simulink model "TBS_SIM"  (R2021a)
settings: Solver=ode5  StartTime=15  StopTime=100  FixedStep=0.002  RelTol=1e-3
PreLoadFcn:
  | TBS_Cai_simu_init_20170316
StopFcn:
  | TBS_SIMULATION_LOG
undefined symbols (not defined in the file): air_density, g, L1X, L2X, L2Y, L3X, L3Y, MAC1, MAC2, MAC3, magnitude, mass, motor_m0, motor_t0, ORIGIN_CD, ORIGIN_CL, ORIGIN_CM, S_seg1, S_seg2, S_seg3
libraries: aerolibconvert2 x20, pid_lib x10, sharedtransform x4, aerolibwind2 x3, simulink x2, shared6dof x1, aerolibasang x1
(part 2 of 3)

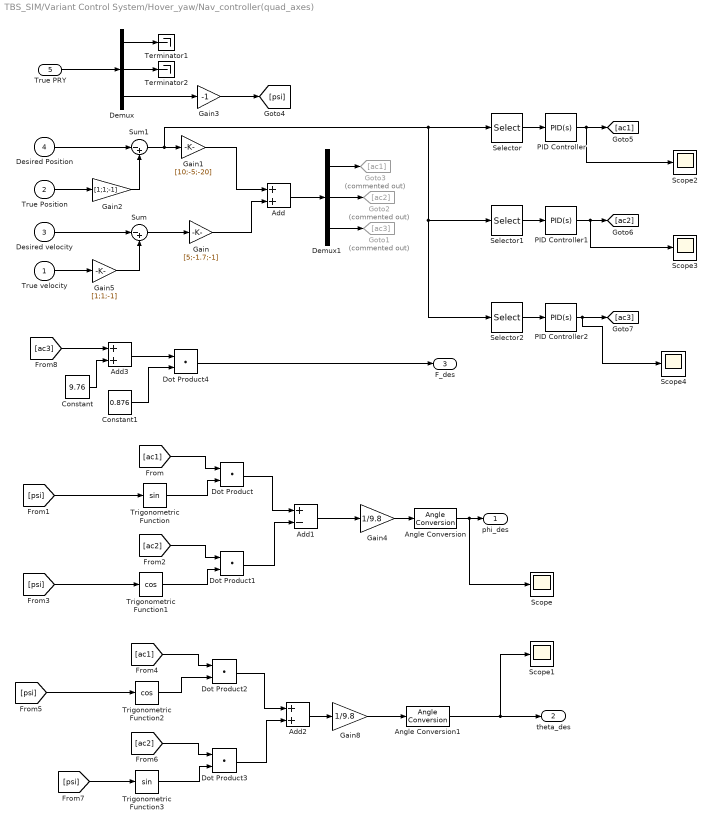
== system TBS_SIM/Variant Control System/Hover_yaw/Nav_controller(quad_axes) ==
  True velocity : Inport
  True Position : Inport  Port=2
  Desired velocity : Inport  Port=3
  Desired Position : Inport  Port=4
  True PRY : Inport  Port=5
  Add : Sum
  Add1 : Sum  Inputs=+-
  Add2 : Sum
  Add3 : Sum
  Angle Conversion : aerolibconvert2/Angle Conversion  IU=rad  OU=deg
  Angle Conversion1 : aerolibconvert2/Angle Conversion  IU=rad  OU=deg
  Constant : Constant  Value=9.76
  Constant1 : Constant  Value=0.876
  Demux : Demux  Outputs=3
  Demux1 : Demux  Outputs=3
  Dot Product{,1..4} (5 alike) : DotProduct  InputSameDT=on  OutDataTypeStr=Inherit: Inherit via internal rule
  Gain : Gain  Gain=[5;-1.7;-1]
  Gain1 : Gain  Gain=[10;-5;-20]
  Gain2 : Gain  Gain=[1;1;-1]
  Gain3 : Gain  Gain=-1
  Gain4 : Gain  Gain=1/9.8
  Gain5 : Gain  Gain=[1;1;-1]
  Gain8 : Gain  Gain=1/9.8
  Goto1 : Goto  Commented=on  GotoTag=ac3
  Goto2 : Goto  Commented=on  GotoTag=ac2
  Goto3 : Goto  Commented=on  GotoTag=ac1
  PID Controller : pid_lib/PID Controller  Controller=PID  Form=Parallel  TimeDomain=Continuous-time  UseExternalTs=off  SampleTime=-1  IntegratorMethod=Forward Euler  FilterMethod=Forward Euler  ControllerParametersSource=internal  P=4  I=3  D=3  UseFilter=on  N=100  TunerSelectOption=Transfer Function Based (PID Tuner App)  InitialConditionSource=internal  InitialConditionForIntegrator=0  InitialConditionForFilter=0  DifferentiatorICPrevScaledInput=0  ExternalReset=none  TrackingMode=off  Kt=1  LimitOutput=off  SatLimitsSource=internal  UpperSaturationLimit=inf  LowerSaturationLimit=-inf  LinearizeAsGain=on  AntiWindupMode=none  Kb=1  POutMin=[]  POutMax=[]  IOutMin=[]  IOutMax=[]  DOutMin=[]  DOutMax=[]  NOutMin=[]  NOutMax=[]  SumOutMin=[]  SumOutMax=[]  SaturationOutMin=[]  SaturationOutMax=[]  PParamMin=[]  PParamMax=[]  IParamMin=[]  IParamMax=[]  DParamMin=[]  DParamMax=[]  NParamMin=[]  NParamMax=[]  KbParamMin=[]  KbParamMax=[]  KtParamMin=[]  KtParamMax=[]  KbOutMin=[]  KbOutMax=[]  KtOutMin=[]  KtOutMax=[]  IntegratorOutMin=[]  IntegratorOutMax=[]  FilterOutMin=[]  FilterOutMax=[]  SumI1OutMin=[]  SumI1OutMax=[]  SumI2OutMin=[]  SumI2OutMax=[]  SumI3OutMin=[]  SumI3OutMax=[]  SumI4OutMin=[]  SumI4OutMax=[]  SumDOutMin=[]  SumDOutMax=[]  DifferentiatorOutMin=[]  DifferentiatorOutMax=[]  FilterDiffOutCoefMin=[]  FilterDiffOutCoefMax=[]  ReciprocalOutMin=[]  ReciprocalOutMax=[]  SumDenOutMin=[]  SumDenOutMax=[]  SumNumOutMin=[]  SumNumOutMax=[]  DivideOutMin=[]  DivideOutMax=[]  UdiffTsProdOutMin=[]  UdiffTsProdOutMax=[]  NTsProdOutMin=[]  NTsProdOutMax=[]  UintegralTsProdOutMin=[]  UintegralTsProdOutMax=[]  UngainTsProdOutMin=[]  UngainTsProdOutMax=[]  IntegratorContinuousStateAttributes=''  IntegratorStateMustResolveToSignalObject=off  IntegratorRTWStateStorageClass=Auto  FilterContinuousStateAttributes=''  FilterStateMustResolveToSignalObject=off  FilterRTWStateStorageClass=Auto  ParallelPVariant=InternalParameters  IdealPVariant=Disabled  IVariant=InternalParameters  DVariant=InternalParameters  IntegratorVariant=Continuous  SatVariant=Disabled  AWVariant=Passthrough  PCopyVariant=Disabled  TRVariant=Disabled  FdbkBlocksVariant=Forward  IdealPFdbkVariant=Disabled  SatFdbkVariant=Disabled  DerivativeFilterVariant=ContFilter  NVariant=InternalParameters  NCopyVariant=Disabled  FilterICVariant=InternalICsFilter  IntegratorICVariant=InternalICs  ExternalResetVariant=Disabled  TRSumVariant=Passthrough  SumFdbkVariant=Disabled  SumVariant=Sum_PID  TsampFilterVariant=InternalTs  TsampNgainVariant=Passthrough  TsampIntegralVariant=Passthrough  ExternalSaturationOutDataTypeStr=Inherit: Same as second input
  PID Controller1 : pid_lib/PID Controller  Controller=PID  Form=Parallel  TimeDomain=Continuous-time  UseExternalTs=off  SampleTime=-1  IntegratorMethod=Forward Euler  FilterMethod=Forward Euler  ControllerParametersSource=internal  P=-8  I=-4  D=-2  UseFilter=on  N=100  TunerSelectOption=Transfer Function Based (PID Tuner App)  InitialConditionSource=internal  InitialConditionForIntegrator=0  InitialConditionForFilter=0  DifferentiatorICPrevScaledInput=0  ExternalReset=none  TrackingMode=off  Kt=1  LimitOutput=off  SatLimitsSource=internal  UpperSaturationLimit=inf  LowerSaturationLimit=-inf  LinearizeAsGain=on  AntiWindupMode=none  Kb=1  POutMin=[]  POutMax=[]  IOutMin=[]  IOutMax=[]  DOutMin=[]  DOutMax=[]  NOutMin=[]  NOutMax=[]  SumOutMin=[]  SumOutMax=[]  SaturationOutMin=[]  SaturationOutMax=[]  PParamMin=[]  PParamMax=[]  IParamMin=[]  IParamMax=[]  DParamMin=[]  DParamMax=[]  NParamMin=[]  NParamMax=[]  KbParamMin=[]  KbParamMax=[]  KtParamMin=[]  KtParamMax=[]  KbOutMin=[]  KbOutMax=[]  KtOutMin=[]  KtOutMax=[]  IntegratorOutMin=[]  IntegratorOutMax=[]  FilterOutMin=[]  FilterOutMax=[]  SumI1OutMin=[]  SumI1OutMax=[]  SumI2OutMin=[]  SumI2OutMax=[]  SumI3OutMin=[]  SumI3OutMax=[]  SumI4OutMin=[]  SumI4OutMax=[]  SumDOutMin=[]  SumDOutMax=[]  DifferentiatorOutMin=[]  DifferentiatorOutMax=[]  FilterDiffOutCoefMin=[]  FilterDiffOutCoefMax=[]  ReciprocalOutMin=[]  ReciprocalOutMax=[]  SumDenOutMin=[]  SumDenOutMax=[]  SumNumOutMin=[]  SumNumOutMax=[]  DivideOutMin=[]  DivideOutMax=[]  UdiffTsProdOutMin=[]  UdiffTsProdOutMax=[]  NTsProdOutMin=[]  NTsProdOutMax=[]  UintegralTsProdOutMin=[]  UintegralTsProdOutMax=[]  UngainTsProdOutMin=[]  UngainTsProdOutMax=[]  IntegratorContinuousStateAttributes=''  IntegratorStateMustResolveToSignalObject=off  IntegratorRTWStateStorageClass=Auto  FilterContinuousStateAttributes=''  FilterStateMustResolveToSignalObject=off  FilterRTWStateStorageClass=Auto  ParallelPVariant=InternalParameters  IdealPVariant=Disabled  IVariant=InternalParameters  DVariant=InternalParameters  IntegratorVariant=Continuous  SatVariant=Disabled  AWVariant=Passthrough  PCopyVariant=Disabled  TRVariant=Disabled  FdbkBlocksVariant=Forward  IdealPFdbkVariant=Disabled  SatFdbkVariant=Disabled  DerivativeFilterVariant=ContFilter  NVariant=InternalParameters  NCopyVariant=Disabled  FilterICVariant=InternalICsFilter  IntegratorICVariant=InternalICs  ExternalResetVariant=Disabled  TRSumVariant=Passthrough  SumFdbkVariant=Disabled  SumVariant=Sum_PID  TsampFilterVariant=InternalTs  TsampNgainVariant=Passthrough  TsampIntegralVariant=Passthrough  ExternalSaturationOutDataTypeStr=Inherit: Same as second input
  PID Controller2 : pid_lib/PID Controller  Controller=PID  Form=Parallel  TimeDomain=Continuous-time  UseExternalTs=off  SampleTime=-1  IntegratorMethod=Forward Euler  FilterMethod=Forward Euler  ControllerParametersSource=internal  P=-9  I=-5  D=-2  UseFilter=on  N=100  TunerSelectOption=Transfer Function Based (PID Tuner App)  InitialConditionSource=internal  InitialConditionForIntegrator=0  InitialConditionForFilter=0  DifferentiatorICPrevScaledInput=0  ExternalReset=none  TrackingMode=off  Kt=1  LimitOutput=off  SatLimitsSource=internal  UpperSaturationLimit=inf  LowerSaturationLimit=-inf  LinearizeAsGain=on  AntiWindupMode=none  Kb=1  POutMin=[]  POutMax=[]  IOutMin=[]  IOutMax=[]  DOutMin=[]  DOutMax=[]  NOutMin=[]  NOutMax=[]  SumOutMin=[]  SumOutMax=[]  SaturationOutMin=[]  SaturationOutMax=[]  PParamMin=[]  PParamMax=[]  IParamMin=[]  IParamMax=[]  DParamMin=[]  DParamMax=[]  NParamMin=[]  NParamMax=[]  KbParamMin=[]  KbParamMax=[]  KtParamMin=[]  KtParamMax=[]  KbOutMin=[]  KbOutMax=[]  KtOutMin=[]  KtOutMax=[]  IntegratorOutMin=[]  IntegratorOutMax=[]  FilterOutMin=[]  FilterOutMax=[]  SumI1OutMin=[]  SumI1OutMax=[]  SumI2OutMin=[]  SumI2OutMax=[]  SumI3OutMin=[]  SumI3OutMax=[]  SumI4OutMin=[]  SumI4OutMax=[]  SumDOutMin=[]  SumDOutMax=[]  DifferentiatorOutMin=[]  DifferentiatorOutMax=[]  FilterDiffOutCoefMin=[]  FilterDiffOutCoefMax=[]  ReciprocalOutMin=[]  ReciprocalOutMax=[]  SumDenOutMin=[]  SumDenOutMax=[]  SumNumOutMin=[]  SumNumOutMax=[]  DivideOutMin=[]  DivideOutMax=[]  UdiffTsProdOutMin=[]  UdiffTsProdOutMax=[]  NTsProdOutMin=[]  NTsProdOutMax=[]  UintegralTsProdOutMin=[]  UintegralTsProdOutMax=[]  UngainTsProdOutMin=[]  UngainTsProdOutMax=[]  IntegratorContinuousStateAttributes=''  IntegratorStateMustResolveToSignalObject=off  IntegratorRTWStateStorageClass=Auto  FilterContinuousStateAttributes=''  FilterStateMustResolveToSignalObject=off  FilterRTWStateStorageClass=Auto  ParallelPVariant=InternalParameters  IdealPVariant=Disabled  IVariant=InternalParameters  DVariant=InternalParameters  IntegratorVariant=Continuous  SatVariant=Disabled  AWVariant=Passthrough  PCopyVariant=Disabled  TRVariant=Disabled  FdbkBlocksVariant=Forward  IdealPFdbkVariant=Disabled  SatFdbkVariant=Disabled  DerivativeFilterVariant=ContFilter  NVariant=InternalParameters  NCopyVariant=Disabled  FilterICVariant=InternalICsFilter  IntegratorICVariant=InternalICs  ExternalResetVariant=Disabled  TRSumVariant=Passthrough  SumFdbkVariant=Disabled  SumVariant=Sum_PID  TsampFilterVariant=InternalTs  TsampNgainVariant=Passthrough  TsampIntegralVariant=Passthrough  ExternalSaturationOutDataTypeStr=Inherit: Same as second input
  Scope{,1..4} (5 alike) : Scope
  Selector : Selector  InputPortWidth=3  IndexOptions=Index vector (dialog)  Indices=[1]  OutputSizes=1
  Selector1 : Selector  InputPortWidth=3  IndexOptions=Index vector (dialog)  Indices=[2]  OutputSizes=1
  Selector2 : Selector  InputPortWidth=3  IndexOptions=Index vector (dialog)  Indices=[3]  OutputSizes=1
  Sum : Sum  Inputs=|-+
  Sum1 : Sum  Inputs=|-+
  Terminator1 : Terminator
  Terminator2 : Terminator
  Trigonometric Function : Trigonometry
  Trigonometric Function1 : Trigonometry  Operator=cos
  Trigonometric Function2 : Trigonometry  Operator=cos
  Trigonometric Function3 : Trigonometry
  phi_des : Outport
  "theta_des " : Outport  Port=2
  F_des : Outport  Port=3
  wires:
  True velocity/1 -> Gain5/1
  Desired velocity/1 -> Sum/1
  Sum/1 -> Gain/1
  Gain1/1 -> Add/1
  Gain/1 -> Add/2
  True PRY/1 -> Demux/1
  Demux/1 -> Terminator1/1
  Demux/3 -> Gain3/1
  Demux/2 -> Terminator2/1
  Add/1 -> Demux1/1
  Demux1/2 -> Goto2/1
  [ac1] -> Dot Product/1
  Trigonometric Function/1 -> Dot Product/2
  [psi] -> Trigonometric Function/1
  [ac2] -> Dot Product1/1
  Trigonometric Function1/1 -> Dot Product1/2
  [psi] -> Trigonometric Function1/1
  Dot Product/1 -> Add1/1
  Dot Product1/1 -> Add1/2
  Add1/1 -> Gain4/1
  [ac1] -> Dot Product2/1
  Trigonometric Function2/1 -> Dot Product2/2
  [psi] -> Trigonometric Function2/1
  [ac2] -> Dot Product3/1
  Trigonometric Function3/1 -> Dot Product3/2
  [psi] -> Trigonometric Function3/1
  Dot Product2/1 -> Add2/1
  Dot Product3/1 -> Add2/2
  Add2/1 -> Gain8/1
  [ac3] -> Add3/1
  Constant/1 -> Add3/2
  Add3/1 -> Dot Product4/1
  Constant1/1 -> Dot Product4/2
  Dot Product4/1 -> F_des/1
  Demux1/1 -> Goto3/1
  Demux1/3 -> Goto1/1
  True Position/1 -> Gain2/1
  Gain2/1 -> Sum1/2
  Desired Position/1 -> Sum1/1
  Gain3/1 -> [psi]
  Gain4/1 -> Angle Conversion/1
  Angle Conversion/1 -> Scope/1, phi_des/1
  Gain8/1 -> Angle Conversion1/1
  Angle Conversion1/1 -> Scope1/1, "theta_des "/1
  Gain5/1 -> Sum/2
  Selector/1 -> PID Controller/1
  PID Controller/1 -> Scope2/1, [ac1]
  Selector1/1 -> PID Controller1/1
  PID Controller1/1 -> Scope3/1, [ac2]
  Sum1/1 -> Selector2/1, Selector1/1, Selector/1, Gain1/1
  Selector2/1 -> PID Controller2/1
  PID Controller2/1 -> Scope4/1, [ac3]

== system TBS_SIM/Variant Control System/Hover_yaw/map1 ==
  F_c : Inport
  M_c : Inport  Port=2
  Constant : Constant  Value=100
  Constant1 : Constant  Value=9.5
  Constant2 : Constant  Value=0.3
  Demux : Demux  Outputs=3
  Gain : Gain  Gain=1000
  Gain1 : Gain  Gain=1000
  Gain2 : Gain  Gain=50
  Gain3 : Gain  Gain=50
  Mux : Mux
  Sum : Sum  Inputs=-+|
  Sum1 : Sum  Inputs=|++
  Sum2 : Sum  Inputs=|+-
  Sum3 : Sum  Inputs=-+|
  Sum4 : Sum  Inputs=|++
  Sum5 : Sum  Inputs=|++
  Sum6 : Sum  Inputs=+-|
  Act : Outport
  wires:
  M_c/1 -> Demux/1
  F_c/1 -> Gain/1
  Demux/1 -> Gain1/1
  Gain1/1 -> Sum/2
  Constant/1 -> Sum/1
  Gain/1 -> Sum2/1, Sum1/1
  Sum/1 -> Sum1/2, Sum2/2
  Sum1/1 -> Mux/1
  Sum2/1 -> Mux/2
  Demux/2 -> Gain2/1
  Demux/3 -> Gain3/1
  Gain3/1 -> Sum4/1
  Constant1/1 -> Sum3/1
  Gain2/1 -> Sum3/2
  Constant2/1 -> Sum4/2
  Mux/1 -> Act/1
  Sum3/1 -> Sum5/1
  Sum4/1 -> Sum6/2, Sum5/2
  Sum5/1 -> Mux/4, Sum6/1
  Sum6/1 -> Mux/3

== system TBS_SIM/Variant Control System/PIDcruise/Subsystem ==
  Euler : Inport
  Constant : Constant  Value=0
  Constant1 : Constant  Value=8
  Constant2 : Constant  Value=0
  Demux : Demux  Outputs=3
  Mux : Mux  Inputs=3
  PID Controller : pid_lib/PID Controller  Controller=PID  Form=Parallel  TimeDomain=Continuous-time  UseExternalTs=off  SampleTime=-1  IntegratorMethod=Forward Euler  FilterMethod=Forward Euler  ControllerParametersSource=internal  P=0.5  I=0.1  D=0.01  UseFilter=on  N=100  TunerSelectOption=Transfer Function Based (PID Tuner App)  InitialConditionSource=internal  InitialConditionForIntegrator=0  InitialConditionForFilter=0  DifferentiatorICPrevScaledInput=0  ExternalReset=none  TrackingMode=off  Kt=1  LimitOutput=off  SatLimitsSource=internal  UpperSaturationLimit=inf  LowerSaturationLimit=-inf  LinearizeAsGain=on  AntiWindupMode=none  Kb=1  POutMin=[]  POutMax=[]  IOutMin=[]  IOutMax=[]  DOutMin=[]  DOutMax=[]  NOutMin=[]  NOutMax=[]  SumOutMin=[]  SumOutMax=[]  SaturationOutMin=[]  SaturationOutMax=[]  PParamMin=[]  PParamMax=[]  IParamMin=[]  IParamMax=[]  DParamMin=[]  DParamMax=[]  NParamMin=[]  NParamMax=[]  KbParamMin=[]  KbParamMax=[]  KtParamMin=[]  KtParamMax=[]  KbOutMin=[]  KbOutMax=[]  KtOutMin=[]  KtOutMax=[]  IntegratorOutMin=[]  IntegratorOutMax=[]  FilterOutMin=[]  FilterOutMax=[]  SumI1OutMin=[]  SumI1OutMax=[]  SumI2OutMin=[]  SumI2OutMax=[]  SumI3OutMin=[]  SumI3OutMax=[]  SumI4OutMin=[]  SumI4OutMax=[]  SumDOutMin=[]  SumDOutMax=[]  DifferentiatorOutMin=[]  DifferentiatorOutMax=[]  FilterDiffOutCoefMin=[]  FilterDiffOutCoefMax=[]  ReciprocalOutMin=[]  ReciprocalOutMax=[]  SumDenOutMin=[]  SumDenOutMax=[]  SumNumOutMin=[]  SumNumOutMax=[]  DivideOutMin=[]  DivideOutMax=[]  UdiffTsProdOutMin=[]  UdiffTsProdOutMax=[]  NTsProdOutMin=[]  NTsProdOutMax=[]  UintegralTsProdOutMin=[]  UintegralTsProdOutMax=[]  UngainTsProdOutMin=[]  UngainTsProdOutMax=[]  IntegratorContinuousStateAttributes=''  IntegratorStateMustResolveToSignalObject=off  IntegratorRTWStateStorageClass=Auto  FilterContinuousStateAttributes=''  FilterStateMustResolveToSignalObject=off  FilterRTWStateStorageClass=Auto  ParallelPVariant=InternalParameters  IdealPVariant=Disabled  IVariant=InternalParameters  DVariant=InternalParameters  IntegratorVariant=Continuous  SatVariant=Disabled  AWVariant=Passthrough  PCopyVariant=Disabled  TRVariant=Disabled  FdbkBlocksVariant=Forward  IdealPFdbkVariant=Disabled  SatFdbkVariant=Disabled  DerivativeFilterVariant=ContFilter  NVariant=InternalParameters  NCopyVariant=Disabled  FilterICVariant=InternalICsFilter  IntegratorICVariant=InternalICs  ExternalResetVariant=Disabled  TRSumVariant=Passthrough  SumFdbkVariant=Disabled  SumVariant=Sum_PID  TsampFilterVariant=InternalTs  TsampNgainVariant=Passthrough  TsampIntegralVariant=Passthrough  ExternalSaturationOutDataTypeStr=Inherit: Same as second input
  PID Controller1 : pid_lib/PID Controller  Controller=PID  Form=Parallel  TimeDomain=Continuous-time  UseExternalTs=off  SampleTime=-1  IntegratorMethod=Forward Euler  FilterMethod=Forward Euler  ControllerParametersSource=internal  P=0.8  I=0.5  D=0.005  UseFilter=on  N=100  TunerSelectOption=Transfer Function Based (PID Tuner App)  InitialConditionSource=internal  InitialConditionForIntegrator=0  InitialConditionForFilter=0  DifferentiatorICPrevScaledInput=0  ExternalReset=none  TrackingMode=off  Kt=1  LimitOutput=off  SatLimitsSource=internal  UpperSaturationLimit=inf  LowerSaturationLimit=-inf  LinearizeAsGain=on  AntiWindupMode=none  Kb=1  POutMin=[]  POutMax=[]  IOutMin=[]  IOutMax=[]  DOutMin=[]  DOutMax=[]  NOutMin=[]  NOutMax=[]  SumOutMin=[]  SumOutMax=[]  SaturationOutMin=[]  SaturationOutMax=[]  PParamMin=[]  PParamMax=[]  IParamMin=[]  IParamMax=[]  DParamMin=[]  DParamMax=[]  NParamMin=[]  NParamMax=[]  KbParamMin=[]  KbParamMax=[]  KtParamMin=[]  KtParamMax=[]  KbOutMin=[]  KbOutMax=[]  KtOutMin=[]  KtOutMax=[]  IntegratorOutMin=[]  IntegratorOutMax=[]  FilterOutMin=[]  FilterOutMax=[]  SumI1OutMin=[]  SumI1OutMax=[]  SumI2OutMin=[]  SumI2OutMax=[]  SumI3OutMin=[]  SumI3OutMax=[]  SumI4OutMin=[]  SumI4OutMax=[]  SumDOutMin=[]  SumDOutMax=[]  DifferentiatorOutMin=[]  DifferentiatorOutMax=[]  FilterDiffOutCoefMin=[]  FilterDiffOutCoefMax=[]  ReciprocalOutMin=[]  ReciprocalOutMax=[]  SumDenOutMin=[]  SumDenOutMax=[]  SumNumOutMin=[]  SumNumOutMax=[]  DivideOutMin=[]  DivideOutMax=[]  UdiffTsProdOutMin=[]  UdiffTsProdOutMax=[]  NTsProdOutMin=[]  NTsProdOutMax=[]  UintegralTsProdOutMin=[]  UintegralTsProdOutMax=[]  UngainTsProdOutMin=[]  UngainTsProdOutMax=[]  IntegratorContinuousStateAttributes=''  IntegratorStateMustResolveToSignalObject=off  IntegratorRTWStateStorageClass=Auto  FilterContinuousStateAttributes=''  FilterStateMustResolveToSignalObject=off  FilterRTWStateStorageClass=Auto  ParallelPVariant=InternalParameters  IdealPVariant=Disabled  IVariant=InternalParameters  DVariant=InternalParameters  IntegratorVariant=Continuous  SatVariant=Disabled  AWVariant=Passthrough  PCopyVariant=Disabled  TRVariant=Disabled  FdbkBlocksVariant=Forward  IdealPFdbkVariant=Disabled  SatFdbkVariant=Disabled  DerivativeFilterVariant=ContFilter  NVariant=InternalParameters  NCopyVariant=Disabled  FilterICVariant=InternalICsFilter  IntegratorICVariant=InternalICs  ExternalResetVariant=Disabled  TRSumVariant=Passthrough  SumFdbkVariant=Disabled  SumVariant=Sum_PID  TsampFilterVariant=InternalTs  TsampNgainVariant=Passthrough  TsampIntegralVariant=Passthrough  ExternalSaturationOutDataTypeStr=Inherit: Same as second input
  PID Controller2 : pid_lib/PID Controller  Controller=PID  Form=Parallel  TimeDomain=Continuous-time  UseExternalTs=off  SampleTime=-1  IntegratorMethod=Forward Euler  FilterMethod=Forward Euler  ControllerParametersSource=internal  P=3  I=1.5  D=0.5  UseFilter=on  N=100  TunerSelectOption=Transfer Function Based (PID Tuner App)  InitialConditionSource=internal  InitialConditionForIntegrator=0  InitialConditionForFilter=0  DifferentiatorICPrevScaledInput=0  ExternalReset=none  TrackingMode=off  Kt=1  LimitOutput=off  SatLimitsSource=internal  UpperSaturationLimit=inf  LowerSaturationLimit=-inf  LinearizeAsGain=on  AntiWindupMode=none  Kb=1  POutMin=[]  POutMax=[]  IOutMin=[]  IOutMax=[]  DOutMin=[]  DOutMax=[]  NOutMin=[]  NOutMax=[]  SumOutMin=[]  SumOutMax=[]  SaturationOutMin=[]  SaturationOutMax=[]  PParamMin=[]  PParamMax=[]  IParamMin=[]  IParamMax=[]  DParamMin=[]  DParamMax=[]  NParamMin=[]  NParamMax=[]  KbParamMin=[]  KbParamMax=[]  KtParamMin=[]  KtParamMax=[]  KbOutMin=[]  KbOutMax=[]  KtOutMin=[]  KtOutMax=[]  IntegratorOutMin=[]  IntegratorOutMax=[]  FilterOutMin=[]  FilterOutMax=[]  SumI1OutMin=[]  SumI1OutMax=[]  SumI2OutMin=[]  SumI2OutMax=[]  SumI3OutMin=[]  SumI3OutMax=[]  SumI4OutMin=[]  SumI4OutMax=[]  SumDOutMin=[]  SumDOutMax=[]  DifferentiatorOutMin=[]  DifferentiatorOutMax=[]  FilterDiffOutCoefMin=[]  FilterDiffOutCoefMax=[]  ReciprocalOutMin=[]  ReciprocalOutMax=[]  SumDenOutMin=[]  SumDenOutMax=[]  SumNumOutMin=[]  SumNumOutMax=[]  DivideOutMin=[]  DivideOutMax=[]  UdiffTsProdOutMin=[]  UdiffTsProdOutMax=[]  NTsProdOutMin=[]  NTsProdOutMax=[]  UintegralTsProdOutMin=[]  UintegralTsProdOutMax=[]  UngainTsProdOutMin=[]  UngainTsProdOutMax=[]  IntegratorContinuousStateAttributes=''  IntegratorStateMustResolveToSignalObject=off  IntegratorRTWStateStorageClass=Auto  FilterContinuousStateAttributes=''  FilterStateMustResolveToSignalObject=off  FilterRTWStateStorageClass=Auto  ParallelPVariant=InternalParameters  IdealPVariant=Disabled  IVariant=InternalParameters  DVariant=InternalParameters  IntegratorVariant=Continuous  SatVariant=Disabled  AWVariant=Passthrough  PCopyVariant=Disabled  TRVariant=Disabled  FdbkBlocksVariant=Forward  IdealPFdbkVariant=Disabled  SatFdbkVariant=Disabled  DerivativeFilterVariant=ContFilter  NVariant=InternalParameters  NCopyVariant=Disabled  FilterICVariant=InternalICsFilter  IntegratorICVariant=InternalICs  ExternalResetVariant=Disabled  TRSumVariant=Passthrough  SumFdbkVariant=Disabled  SumVariant=Sum_PID  TsampFilterVariant=InternalTs  TsampNgainVariant=Passthrough  TsampIntegralVariant=Passthrough  ExternalSaturationOutDataTypeStr=Inherit: Same as second input
  Sum : Sum  Inputs=+-|
  Sum1 : Sum  Inputs=+-|
  Sum2 : Sum  Inputs=+-|
  Out1 : Outport
  wires:
  Euler/1 -> Demux/1
  Sum/1 -> PID Controller/1
  Demux/1 -> Sum/2
  Constant/1 -> Sum/1
  Sum1/1 -> PID Controller1/1
  Demux/2 -> Sum1/2
  Constant1/1 -> Sum1/1
  Sum2/1 -> PID Controller2/1
  Demux/3 -> Sum2/2
  Constant2/1 -> Sum2/1
  PID Controller/1 -> Mux/1
  PID Controller1/1 -> Mux/2
  PID Controller2/1 -> Mux/3
  Mux/1 -> Out1/1

== system TBS_SIM/Variant Control System/PIDcruise/Subsystem1 ==
  Velocity : Inport
  Constant : Constant  Value=10
  PID Controller2 : pid_lib/PID Controller  Controller=PID  Form=Parallel  TimeDomain=Continuous-time  UseExternalTs=off  SampleTime=-1  IntegratorMethod=Forward Euler  FilterMethod=Forward Euler  ControllerParametersSource=internal  P=3  I=1  D=0.5  UseFilter=on  N=100  TunerSelectOption=Transfer Function Based (PID Tuner App)  InitialConditionSource=internal  InitialConditionForIntegrator=0  InitialConditionForFilter=0  DifferentiatorICPrevScaledInput=0  ExternalReset=none  TrackingMode=off  Kt=1  LimitOutput=off  SatLimitsSource=internal  UpperSaturationLimit=inf  LowerSaturationLimit=-inf  LinearizeAsGain=on  AntiWindupMode=none  Kb=1  POutMin=[]  POutMax=[]  IOutMin=[]  IOutMax=[]  DOutMin=[]  DOutMax=[]  NOutMin=[]  NOutMax=[]  SumOutMin=[]  SumOutMax=[]  SaturationOutMin=[]  SaturationOutMax=[]  PParamMin=[]  PParamMax=[]  IParamMin=[]  IParamMax=[]  DParamMin=[]  DParamMax=[]  NParamMin=[]  NParamMax=[]  KbParamMin=[]  KbParamMax=[]  KtParamMin=[]  KtParamMax=[]  KbOutMin=[]  KbOutMax=[]  KtOutMin=[]  KtOutMax=[]  IntegratorOutMin=[]  IntegratorOutMax=[]  FilterOutMin=[]  FilterOutMax=[]  SumI1OutMin=[]  SumI1OutMax=[]  SumI2OutMin=[]  SumI2OutMax=[]  SumI3OutMin=[]  SumI3OutMax=[]  SumI4OutMin=[]  SumI4OutMax=[]  SumDOutMin=[]  SumDOutMax=[]  DifferentiatorOutMin=[]  DifferentiatorOutMax=[]  FilterDiffOutCoefMin=[]  FilterDiffOutCoefMax=[]  ReciprocalOutMin=[]  ReciprocalOutMax=[]  SumDenOutMin=[]  SumDenOutMax=[]  SumNumOutMin=[]  SumNumOutMax=[]  DivideOutMin=[]  DivideOutMax=[]  UdiffTsProdOutMin=[]  UdiffTsProdOutMax=[]  NTsProdOutMin=[]  NTsProdOutMax=[]  UintegralTsProdOutMin=[]  UintegralTsProdOutMax=[]  UngainTsProdOutMin=[]  UngainTsProdOutMax=[]  IntegratorContinuousStateAttributes=''  IntegratorStateMustResolveToSignalObject=off  IntegratorRTWStateStorageClass=Auto  FilterContinuousStateAttributes=''  FilterStateMustResolveToSignalObject=off  FilterRTWStateStorageClass=Auto  ParallelPVariant=InternalParameters  IdealPVariant=Disabled  IVariant=InternalParameters  DVariant=InternalParameters  IntegratorVariant=Continuous  SatVariant=Disabled  AWVariant=Passthrough  PCopyVariant=Disabled  TRVariant=Disabled  FdbkBlocksVariant=Forward  IdealPFdbkVariant=Disabled  SatFdbkVariant=Disabled  DerivativeFilterVariant=ContFilter  NVariant=InternalParameters  NCopyVariant=Disabled  FilterICVariant=InternalICsFilter  IntegratorICVariant=InternalICs  ExternalResetVariant=Disabled  TRSumVariant=Passthrough  SumFdbkVariant=Disabled  SumVariant=Sum_PID  TsampFilterVariant=InternalTs  TsampNgainVariant=Passthrough  TsampIntegralVariant=Passthrough  ExternalSaturationOutDataTypeStr=Inherit: Same as second input
  Selector : Selector  InputPortWidth=3  IndexOptions=Index vector (dialog)  Indices=[1]  OutputSizes=1
  Sum2 : Sum  Inputs=+-|
  Out1 : Outport
  wires:
  Velocity/1 -> Selector/1
  Sum2/1 -> PID Controller2/1
  PID Controller2/1 -> Out1/1
  Selector/1 -> Sum2/2
  Constant/1 -> Sum2/1

== system TBS_SIM/Variant Control System/PIDcruise/Subsystem2 ==
  Moment : Inport
  Fprce : Inport  Port=2
  Demux : Demux  Outputs=3
  Gain : Gain  Gain=2000
  Gain1 : Gain  Gain=-50
  Gain2 : Gain  Gain=50
  Gain3 : Gain  Gain=-1000
  Mux : Mux
  Sum : Sum  Inputs=++|
  Sum1 : Sum  Inputs=-+|
  Sum2 : Sum  Inputs=2
  Sum3 : Sum  Inputs=-+
  Out1 : Outport
  wires:
  Fprce/1 -> Gain/1
  Moment/1 -> Demux/1
  Demux/2 -> Gain1/1
  Demux/1 -> Gain2/1
  Demux/3 -> Gain3/1
  Gain3/1 -> Sum/1, Sum1/1
  Gain/1 -> Sum1/2, Sum/2
  Sum/1 -> Mux/1
  Sum1/1 -> Mux/2
  Gain2/1 -> Sum3/1, Sum2/1
  Gain1/1 -> Sum3/2, Sum2/2
  Sum2/1 -> Mux/4
  Sum3/1 -> Mux/3
  Mux/1 -> Out1/1

== system TBS_SIM/Variant Control System/Transition/Trans ==
  State : Inport
  Bus Selector : BusSelector  OutputSignals=v_b,euler
  Chart1 : Stateflow chart  TreatAsAtomicUnit=on
  Cruise Controller : Subsystem
  Demux : Demux  Outputs=3
  Demux1 : Demux  Outputs=3
  MATLAB Function : MATLAB Function  TreatAsAtomicUnit=on
  Scope : Scope
  Switch : Switch  Criteria=u2 ~= 0
  Terminator{,1..3} (4 alike) : Terminator
  Transition Controller : Subsystem
  Commands : Outport
  wires:
  Demux1/3 -> Terminator3/1
  Demux1/1 -> Terminator2/1
  Demux/3 -> Terminator1/1
  Demux/2 -> Terminator/1
  Demux1/2 -> MATLAB Function/2(pitch)
  Bus Selector/2 -> Demux1/1  "<euler>"
  Demux/1 -> MATLAB Function/1(v)
  Bus Selector/1 -> Demux/1  "<v_b>"
  Switch/1 -> Commands/1
  State/1 -> Transition Controller/1(state 1), Bus Selector/1, Cruise Controller/1(State)
  Cruise Controller/1("Commands ") -> Switch/3
  Transition Controller/1("Command ") -> Switch/1
  MATLAB Function/1(y) -> Switch/2, Scope/1

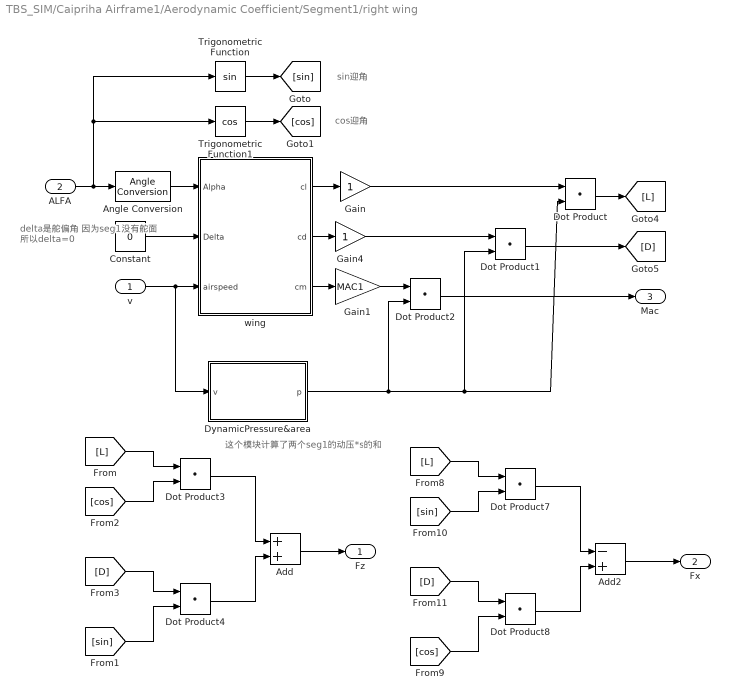
== system TBS_SIM/Caipriha Airframe1/Aerodynamic Coefficient/Segment1/right wing ==
  note: 这个模块计算了两个seg1的动压*s的和
  note: delta是舵偏角
      | 因为seg1没有舵面
      | 所以delta=0
  note: cos迎角
  note: sin迎角
  v : Inport
  "ALFA " : Inport  Port=2
  Add : Sum
  Add2 : Sum  Inputs=-+
  Angle Conversion : aerolibconvert2/Angle Conversion  IU=rad  OU=deg
  Constant : Constant  Value=0
  Dot Product{,1..4,7..8} (7 alike) : DotProduct  InputSameDT=on  OutDataTypeStr=Inherit: Inherit via internal rule
  DynamicPressure&area : Subsystem
  Gain : Gain
  Gain1 : Gain  Gain=MAC1
  Gain4 : Gain
  Trigonometric Function : Trigonometry
  Trigonometric Function1 : Trigonometry  Operator=cos
  wing : Subsystem
  Fz : Outport
  Fx : Outport  Port=2
  Mac : Outport  Port=3
  wires:
  wing/3(cm) -> Gain1/1
  Gain4/1 -> Dot Product1/1
  Gain/1 -> Dot Product/1
  wing/1(cl) -> Gain/1
  v/1 -> DynamicPressure&area/1(v), wing/3(airspeed)
  Constant/1 -> wing/2(Delta)
  DynamicPressure&area/1(p) -> Dot Product/2, Dot Product1/2, Dot Product2/2
  wing/2(cd) -> Gain4/1
  Gain1/1 -> Dot Product2/1
  Dot Product2/1 -> Mac/1
  Angle Conversion/1 -> wing/1(Alpha)
  Trigonometric Function/1 -> [sin]
  "ALFA "/1 -> Trigonometric Function/1, Trigonometric Function1/1, Angle Conversion/1
  Trigonometric Function1/1 -> [cos]
  Dot Product/1 -> [L]
  Dot Product1/1 -> [D]
  [L] -> Dot Product3/1
  [cos] -> Dot Product3/2
  [D] -> Dot Product4/1
  [sin] -> Dot Product4/2
  Dot Product3/1 -> Add/1
  Dot Product4/1 -> Add/2
  Add/1 -> Fz/1
  [L] -> Dot Product7/1
  [sin] -> Dot Product7/2
  [D] -> Dot Product8/1
  [cos] -> Dot Product8/2
  Dot Product7/1 -> Add2/1
  Dot Product8/1 -> Add2/2
  Add2/1 -> Fx/1

== system TBS_SIM/Caipriha Airframe1/Aerodynamic Coefficient/Segment2/immersed velocity ==
  alpha : Inport
  "t1 " : Inport  Port=2
  t2 : Inport  Port=3
  airspeed : Inport  Port=4
  "Immersed velocity " : Subsystem
  Immersed velocity 1 : Subsystem
  v1 : Outport
  v2 : Outport  Port=2
  wires:
  airspeed/1 -> "Immersed velocity "/2(airspeed), Immersed velocity 1/2(airspeed)
  alpha/1 -> Immersed velocity 1/3(alfa), "Immersed velocity "/3(alfa)
  Immersed velocity 1/1(v) -> v2/1
  "Immersed velocity "/1(v) -> v1/1
  t2/1 -> Immersed velocity 1/1(T)
  "t1 "/1 -> "Immersed velocity "/1(T)

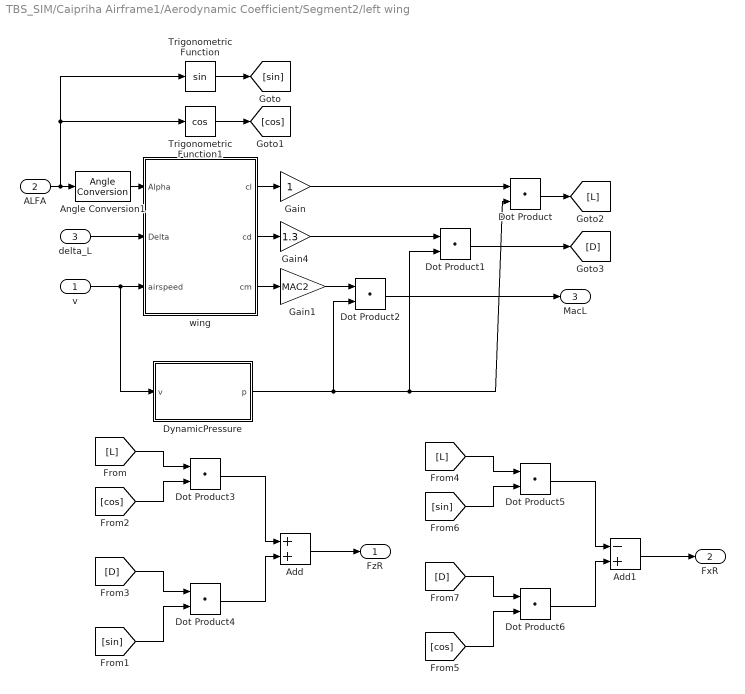
== system TBS_SIM/Caipriha Airframe1/Aerodynamic Coefficient/Segment2/left wing ==
  v : Inport
  "ALFA " : Inport  Port=2
  delta_L : Inport  Port=3
  Add : Sum
  Add1 : Sum  Inputs=-+
  Angle Conversion1 : aerolibconvert2/Angle Conversion  IU=rad  OU=deg
  Dot Product{,1..6} (7 alike) : DotProduct  InputSameDT=on  OutDataTypeStr=Inherit: Inherit via internal rule
  DynamicPressure : Subsystem
  Gain : Gain
  Gain1 : Gain  Gain=MAC2
  Gain4 : Gain  Gain=1.3
  Trigonometric Function : Trigonometry
  Trigonometric Function1 : Trigonometry  Operator=cos
  wing : Subsystem
  FzR : Outport
  FxR : Outport  Port=2
  MacL : Outport  Port=3
  wires:
  wing/3(cm) -> Gain1/1
  Gain4/1 -> Dot Product1/1
  Gain/1 -> Dot Product/1
  wing/1(cl) -> Gain/1
  v/1 -> DynamicPressure/1(v), wing/3(airspeed)
  delta_L/1 -> wing/2(Delta)
  DynamicPressure/1(p) -> Dot Product/2, Dot Product1/2, Dot Product2/2
  wing/2(cd) -> Gain4/1
  Gain1/1 -> Dot Product2/1
  Dot Product2/1 -> MacL/1
  Angle Conversion1/1 -> wing/1(Alpha)
  Trigonometric Function/1 -> [sin]
  "ALFA "/1 -> Trigonometric Function/1, Trigonometric Function1/1, Angle Conversion1/1
  Trigonometric Function1/1 -> [cos]
  Dot Product/1 -> [L]
  Dot Product1/1 -> [D]
  [L] -> Dot Product3/1
  [cos] -> Dot Product3/2
  [D] -> Dot Product4/1
  [sin] -> Dot Product4/2
  Dot Product3/1 -> Add/1
  Dot Product4/1 -> Add/2
  Add/1 -> FzR/1
  [L] -> Dot Product5/1
  [sin] -> Dot Product5/2
  [D] -> Dot Product6/1
  [cos] -> Dot Product6/2
  Dot Product5/1 -> Add1/1
  Dot Product6/1 -> Add1/2
  Add1/1 -> FxR/1

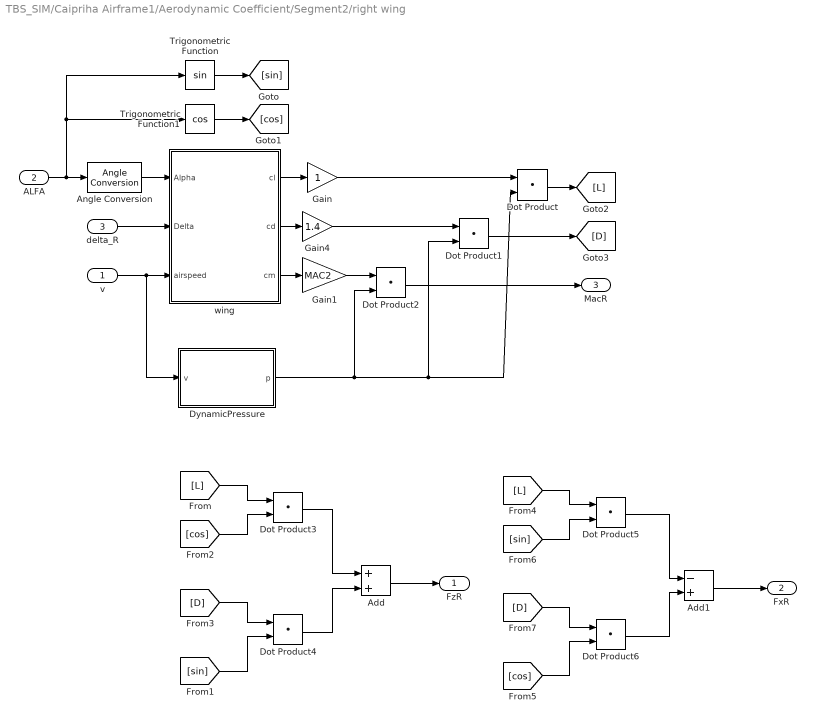
== system TBS_SIM/Caipriha Airframe1/Aerodynamic Coefficient/Segment2/right wing ==
  v : Inport
  "ALFA " : Inport  Port=2
  delta_R : Inport  Port=3
  Add : Sum
  Add1 : Sum  Inputs=-+
  Angle Conversion : aerolibconvert2/Angle Conversion  IU=rad  OU=deg
  Dot Product{,1..6} (7 alike) : DotProduct  InputSameDT=on  OutDataTypeStr=Inherit: Inherit via internal rule
  DynamicPressure : Subsystem
  Gain : Gain
  Gain1 : Gain  Gain=MAC2
  Gain4 : Gain  Gain=1.4
  Trigonometric Function : Trigonometry
  Trigonometric Function1 : Trigonometry  Operator=cos
  wing : Subsystem
  FzR : Outport
  FxR : Outport  Port=2
  MacR : Outport  Port=3
  wires:
  wing/3(cm) -> Gain1/1
  Gain4/1 -> Dot Product1/1
  Gain/1 -> Dot Product/1
  wing/1(cl) -> Gain/1
  v/1 -> DynamicPressure/1(v), wing/3(airspeed)
  delta_R/1 -> wing/2(Delta)
  DynamicPressure/1(p) -> Dot Product/2, Dot Product1/2, Dot Product2/2
  wing/2(cd) -> Gain4/1
  Gain1/1 -> Dot Product2/1
  Dot Product2/1 -> MacR/1
  Angle Conversion/1 -> wing/1(Alpha)
  Trigonometric Function/1 -> [sin]
  "ALFA "/1 -> Trigonometric Function/1, Trigonometric Function1/1, Angle Conversion/1
  Trigonometric Function1/1 -> [cos]
  Dot Product/1 -> [L]
  Dot Product1/1 -> [D]
  [L] -> Dot Product3/1
  [cos] -> Dot Product3/2
  [D] -> Dot Product4/1
  [sin] -> Dot Product4/2
  Dot Product3/1 -> Add/1
  Dot Product4/1 -> Add/2
  Add/1 -> FzR/1
  [L] -> Dot Product5/1
  [sin] -> Dot Product5/2
  [D] -> Dot Product6/1
  [cos] -> Dot Product6/2
  Dot Product5/1 -> Add1/1
  Dot Product6/1 -> Add1/2
  Add1/1 -> FxR/1

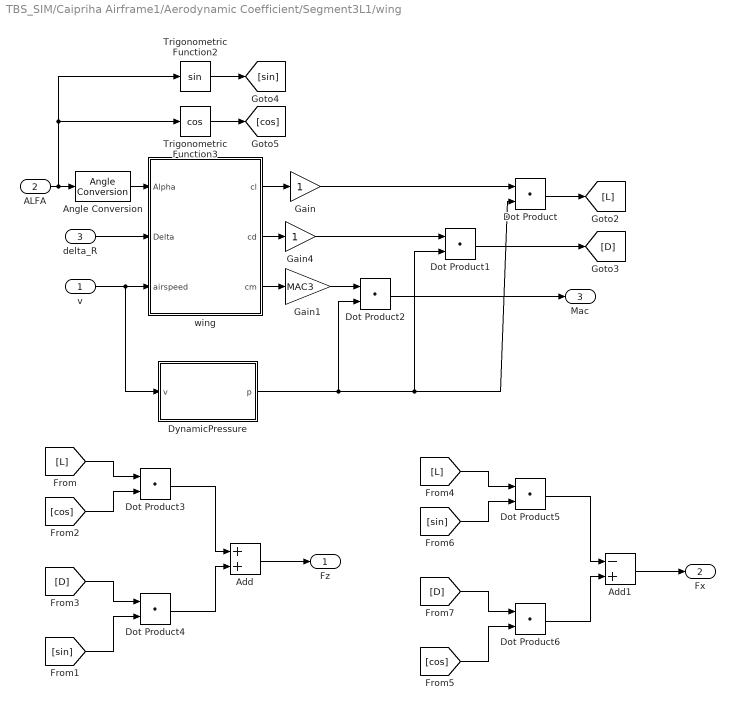
== system TBS_SIM/Caipriha Airframe1/Aerodynamic Coefficient/Segment3L1/wing ==
  v : Inport
  "ALFA " : Inport  Port=2
  delta_R : Inport  Port=3
  Add : Sum
  Add1 : Sum  Inputs=-+
  Angle Conversion : aerolibconvert2/Angle Conversion  IU=rad  OU=deg
  Dot Product{,1..6} (7 alike) : DotProduct  InputSameDT=on  OutDataTypeStr=Inherit: Inherit via internal rule
  DynamicPressure : Subsystem
  Gain : Gain
  Gain1 : Gain  Gain=MAC3
  Gain4 : Gain
  Trigonometric Function2 : Trigonometry
  Trigonometric Function3 : Trigonometry  Operator=cos
  wing : Subsystem
  Fz : Outport
  Fx : Outport  Port=2
  Mac : Outport  Port=3
  wires:
  wing/3(cm) -> Gain1/1
  Gain4/1 -> Dot Product1/1
  Gain/1 -> Dot Product/1
  wing/1(cl) -> Gain/1
  v/1 -> DynamicPressure/1(v), wing/3(airspeed)
  delta_R/1 -> wing/2(Delta)
  DynamicPressure/1(p) -> Dot Product/2, Dot Product1/2, Dot Product2/2
  wing/2(cd) -> Gain4/1
  Gain1/1 -> Dot Product2/1
  Dot Product2/1 -> Mac/1
  Angle Conversion/1 -> wing/1(Alpha)
  Trigonometric Function2/1 -> [sin]
  "ALFA "/1 -> Trigonometric Function2/1, Trigonometric Function3/1, Angle Conversion/1
  Trigonometric Function3/1 -> [cos]
  Dot Product/1 -> [L]
  Dot Product1/1 -> [D]
  [L] -> Dot Product3/1
  [cos] -> Dot Product3/2
  [D] -> Dot Product4/1
  [sin] -> Dot Product4/2
  Dot Product3/1 -> Add/1
  Dot Product4/1 -> Add/2
  Add/1 -> Fz/1
  [L] -> Dot Product5/1
  [sin] -> Dot Product5/2
  [D] -> Dot Product6/1
  [cos] -> Dot Product6/2
  Dot Product5/1 -> Add1/1
  Dot Product6/1 -> Add1/2
  Add1/1 -> Fx/1

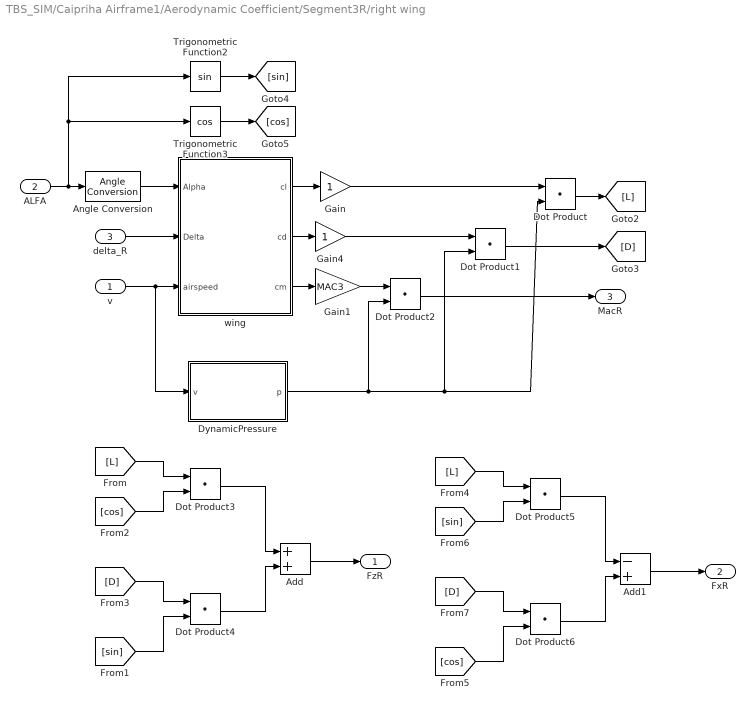
== system TBS_SIM/Caipriha Airframe1/Aerodynamic Coefficient/Segment3R/right wing ==
  v : Inport
  "ALFA " : Inport  Port=2
  delta_R : Inport  Port=3
  Add : Sum
  Add1 : Sum  Inputs=-+
  Angle Conversion : aerolibconvert2/Angle Conversion  IU=rad  OU=deg
  Dot Product{,1..6} (7 alike) : DotProduct  InputSameDT=on  OutDataTypeStr=Inherit: Inherit via internal rule
  DynamicPressure : Subsystem
  Gain : Gain
  Gain1 : Gain  Gain=MAC3
  Gain4 : Gain
  Trigonometric Function2 : Trigonometry
  Trigonometric Function3 : Trigonometry  Operator=cos
  wing : Subsystem
  FzR : Outport
  FxR : Outport  Port=2
  MacR : Outport  Port=3
  wires:
  wing/3(cm) -> Gain1/1
  Gain4/1 -> Dot Product1/1
  Gain/1 -> Dot Product/1
  wing/1(cl) -> Gain/1
  v/1 -> DynamicPressure/1(v), wing/3(airspeed)
  delta_R/1 -> wing/2(Delta)
  DynamicPressure/1(p) -> Dot Product/2, Dot Product1/2, Dot Product2/2
  wing/2(cd) -> Gain4/1
  Gain1/1 -> Dot Product2/1
  Dot Product2/1 -> MacR/1
  Angle Conversion/1 -> wing/1(Alpha)
  Trigonometric Function2/1 -> [sin]
  "ALFA "/1 -> Trigonometric Function2/1, Trigonometric Function3/1, Angle Conversion/1
  Trigonometric Function3/1 -> [cos]
  Dot Product/1 -> [L]
  Dot Product1/1 -> [D]
  [L] -> Dot Product3/1
  [cos] -> Dot Product3/2
  [D] -> Dot Product4/1
  [sin] -> Dot Product4/2
  Dot Product3/1 -> Add/1
  Dot Product4/1 -> Add/2
  Add/1 -> FzR/1
  [L] -> Dot Product5/1
  [sin] -> Dot Product5/2
  [D] -> Dot Product6/1
  [cos] -> Dot Product6/2
  Dot Product5/1 -> Add1/1
  Dot Product6/1 -> Add1/2
  Add1/1 -> FxR/1

== system TBS_SIM/Variant Control System/Transition/Trans/Cruise Controller ==
  State : Inport
  Bus Selector : BusSelector  OutputSignals=v_e,x_e,DCM,omega,v_b,euler
  Cruise : Subsystem  VariantControl=CruseController
  Mux1 : Mux  Inputs=2
  "Commands " : Outport
  wires:
  Mux1/1 -> "Commands "/1
  Bus Selector/6 -> Cruise/6(Euler)  "<euler>"
  State/1 -> Bus Selector/1
  Cruise/1(RS) -> Mux1/1
  Cruise/2("Actuator ") -> Mux1/2
  Bus Selector/5 -> Cruise/5(V_b)  "<v_b>"
  Bus Selector/4 -> Cruise/4(pqr)  "<omega>"
  Bus Selector/3 -> Cruise/3(DCM)  "<DCM>"
  Bus Selector/2 -> Cruise/2(Xe)  "<x_e>"
  Bus Selector/1 -> Cruise/1(Ve)  "<v_e>"

== system TBS_SIM/Variant Control System/Transition/Trans/Transition Controller ==
  state 1 : Inport
  Bus Selector1 : BusSelector  OutputSignals=v_e,x_e,DCM,omega
  Constant : Constant  Value=[0,0,0]
  Constant2 : Constant  Value=0
  Hover : Subsystem  VariantControl=HoveringController
  Mux : Mux  Inputs=3
  Mux2 : Mux  Inputs=2
  Ramp : simulink/Sources/Ramp  slope=0.8  start=1  InitialOutput=0
  Saturation4 : Saturate  UpperLimit=3.5  LowerLimit=0
  "Command " : Outport
  wires:
  Mux2/1 -> "Command "/1
  Hover/2("Actuator ") -> Mux2/2
  Hover/1(RS) -> Mux2/1
  state 1/1 -> Bus Selector1/1
  Bus Selector1/1 -> Hover/1(Ve)  "<v_e>"
  Bus Selector1/2 -> Hover/2(Xe)  "<x_e>"
  Bus Selector1/3 -> Hover/3(DCM)  "<DCM>"
  Bus Selector1/4 -> Hover/4(pqr)  "<omega>"
  Constant/1 -> Hover/6(des_p)
  Mux/1 -> Hover/5(des_v)
  Constant2/1 -> Mux/1, Mux/2
  Saturation4/1 -> Mux/3
  Ramp/1 -> Saturation4/1

== system TBS_SIM/Caipriha Airframe1/Aerodynamic Coefficient/Segment1/right wing/DynamicPressure&area ==
  v : Inport
  Gain1 : Gain  Gain=air_density
  Gain2 : Gain  Gain=0.5
  Gain3 : Gain  Gain=S_seg1*2
  Math Function : Math  Operator=magnitude^2  SignedPower=on  SaturateOnIntegerOverflow=on
  p : Outport
  wires:
  Gain3/1 -> p/1
  Gain2/1 -> Gain3/1
  Gain1/1 -> Gain2/1
  Math Function/1 -> Gain1/1
  v/1 -> Math Function/1

== system TBS_SIM/Caipriha Airframe1/Aerodynamic Coefficient/Segment1/right wing/wing ==
  Alpha : Inport
  Delta : Inport  Port=2
  airspeed : Inport  Port=3
  AirspeedLookup : PreLookup  BreakpointsData=as  BeginIndexSearchUsingPreviousIndexResult=on  ExtrapMethod=Linear
  AlphaLookup : PreLookup  BreakpointsData=alpha_vec_0  BeginIndexSearchUsingPreviousIndexResult=on  ExtrapMethod=Linear
  CD : Interpolation_n-D  NumberOfTableDimensions=3  Table=ORIGIN_CD  ExtrapMethod=Clip  DiagnosticForOutOfRangeInput=Warning  InternalRulePriority=Speed
      settings: InputPortMap=u0,u1,u2,u3,u4,u5
  CD1 : Interpolation_n-D  NumberOfTableDimensions=3  Table=ORIGIN_CM  ExtrapMethod=Clip  DiagnosticForOutOfRangeInput=Warning  InternalRulePriority=Speed
      settings: InputPortMap=u0,u1,u2,u3,u4,u5
  CL : Interpolation_n-D  NumberOfTableDimensions=3  Table=ORIGIN_CL  ExtrapMethod=Clip  DiagnosticForOutOfRangeInput=Warning  InternalRulePriority=Speed
      settings: InputPortMap=u0,u1,u2,u3,u4,u5
  DeltaLookup : PreLookup  BreakpointsData=ORIGIN_DELTA  BeginIndexSearchUsingPreviousIndexResult=on  ExtrapMethod=Linear
  cl : Outport
  cd : Outport  Port=2
  cm : Outport  Port=3
  wires:
  Alpha/1 -> AlphaLookup/1
  airspeed/1 -> AirspeedLookup/1
  DeltaLookup/1 -> CD1/5, CL/5, CD/5
  DeltaLookup/2 -> CD1/6, CL/6, CD/6
  CL/1 -> cl/1
  AirspeedLookup/1 -> CD1/1, CD/1, CL/1
  AirspeedLookup/2 -> CD1/2, CD/2, CL/2
  AlphaLookup/1 -> CD/3, CD1/3, CL/3
  AlphaLookup/2 -> CD1/4, CD/4, CL/4
  CD/1 -> cd/1
  CD1/1 -> cm/1
  Delta/1 -> DeltaLookup/1

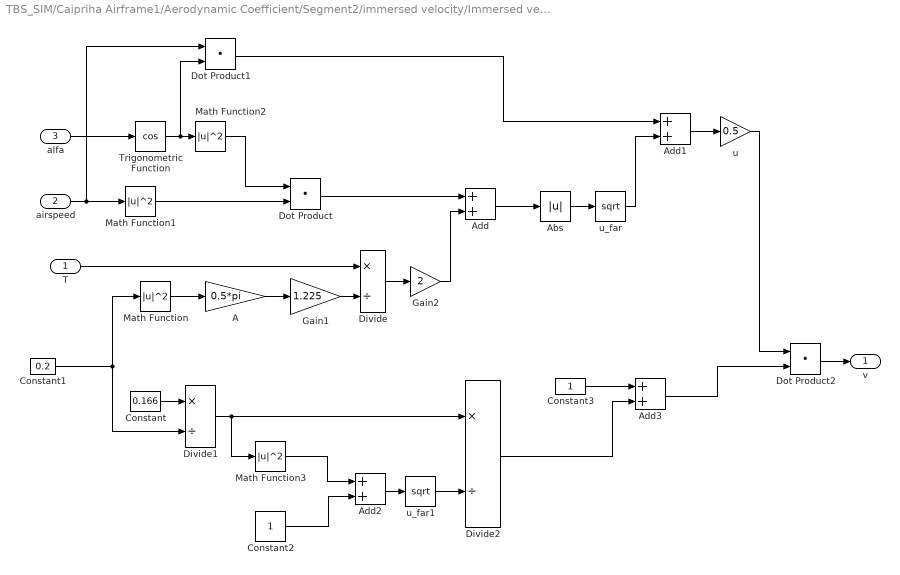
== system TBS_SIM/Caipriha Airframe1/Aerodynamic Coefficient/Segment2/immersed velocity/Immersed velocity  ==
  T : Inport
  airspeed : Inport  Port=2
  alfa : Inport  Port=3
  A : Gain  Gain=0.5*pi
  Abs : Abs
  Add{,1..3} (4 alike) : Sum
  Constant : Constant  Value=0.166
  Constant1 : Constant  Value=0.2
  Constant2 : Constant
  Constant3 : Constant
  Divide : Product  Inputs=*/
  Divide1 : Product  Inputs=*/
  Divide2 : Product  Inputs=*/
  Dot Product : DotProduct  InputSameDT=on  OutDataTypeStr=Inherit: Inherit via internal rule
  Dot Product1 : DotProduct  InputSameDT=on  OutDataTypeStr=Inherit: Inherit via internal rule
  Dot Product2 : DotProduct  InputSameDT=on  OutDataTypeStr=Inherit: Inherit via internal rule
  Gain1 : Gain  Gain=1.225
  Gain2 : Gain  Gain=2
  Math Function{,1..3} (4 alike) : Math  Operator=magnitude^2  SignedPower=on  SaturateOnIntegerOverflow=on
  Trigonometric Function : Trigonometry  Operator=cos
  u : Gain  Gain=0.5
  u_far : Sqrt  SaturateOnIntegerOverflow=on
  u_far1 : Sqrt  SaturateOnIntegerOverflow=on
  v : Outport
  wires:
  Add3/1 -> Dot Product2/2
  Divide2/1 -> Add3/2
  u/1 -> Dot Product2/1
  Constant3/1 -> Add3/1
  Divide1/1 -> Divide2/1, Math Function3/1
  u_far1/1 -> Divide2/2
  Add2/1 -> u_far1/1
  Constant2/1 -> Add2/2
  Math Function3/1 -> Add2/1
  Constant/1 -> Divide1/1
  Add1/1 -> u/1
  Dot Product1/1 -> Add1/1
  u_far/1 -> Add1/2
  Math Function2/1 -> Dot Product/1
  Trigonometric Function/1 -> Math Function2/1, Dot Product1/2
  Abs/1 -> u_far/1
  Add/1 -> Abs/1
  Gain2/1 -> Add/2
  Dot Product/1 -> Add/1
  Math Function1/1 -> Dot Product/2
  alfa/1 -> Trigonometric Function/1
  airspeed/1 -> Math Function1/1, Dot Product1/1
  Divide/1 -> Gain2/1
  T/1 -> Divide/1
  Gain1/1 -> Divide/2
  A/1 -> Gain1/1
  Math Function/1 -> A/1
  Constant1/1 -> Math Function/1, Divide1/2
  Dot Product2/1 -> v/1

== system TBS_SIM/Caipriha Airframe1/Aerodynamic Coefficient/Segment2/immersed velocity/Immersed velocity 1 ==
  T : Inport
  airspeed : Inport  Port=2
  alfa : Inport  Port=3
  A : Gain  Gain=0.5*pi
  Abs : Abs
  Add{,1..3} (4 alike) : Sum
  Constant : Constant  Value=0.166
  Constant1 : Constant  Value=0.2
  Constant2 : Constant
  Constant3 : Constant
  Divide : Product  Inputs=*/
  Divide1 : Product  Inputs=*/
  Divide2 : Product  Inputs=*/
  Dot Product : DotProduct  InputSameDT=on  OutDataTypeStr=Inherit: Inherit via internal rule
  Dot Product1 : DotProduct  InputSameDT=on  OutDataTypeStr=Inherit: Inherit via internal rule
  Dot Product2 : DotProduct  InputSameDT=on  OutDataTypeStr=Inherit: Inherit via internal rule
  Gain1 : Gain  Gain=1.225
  Gain2 : Gain  Gain=2
  Math Function{,1..3} (4 alike) : Math  Operator=magnitude^2  SignedPower=on  SaturateOnIntegerOverflow=on
  Trigonometric Function : Trigonometry  Operator=cos
  u : Gain  Gain=0.5
  u_far : Sqrt  SaturateOnIntegerOverflow=on
  u_far1 : Sqrt  SaturateOnIntegerOverflow=on
  v : Outport
  wires:
  Add3/1 -> Dot Product2/2
  Divide2/1 -> Add3/2
  Constant3/1 -> Add3/1
  Dot Product2/1 -> v/1
  u/1 -> Dot Product2/1
  Divide1/1 -> Math Function3/1, Divide2/1
  u_far1/1 -> Divide2/2
  Add2/1 -> u_far1/1
  Constant2/1 -> Add2/2
  Math Function3/1 -> Add2/1
  Constant/1 -> Divide1/1
  Add1/1 -> u/1
  Dot Product1/1 -> Add1/1
  u_far/1 -> Add1/2
  Math Function2/1 -> Dot Product/1
  Trigonometric Function/1 -> Math Function2/1, Dot Product1/2
  Abs/1 -> u_far/1
  Add/1 -> Abs/1
  Gain2/1 -> Add/2
  Dot Product/1 -> Add/1
  Math Function1/1 -> Dot Product/2
  alfa/1 -> Trigonometric Function/1
  airspeed/1 -> Math Function1/1, Dot Product1/1
  Divide/1 -> Gain2/1
  T/1 -> Divide/1
  Gain1/1 -> Divide/2
  A/1 -> Gain1/1
  Math Function/1 -> A/1
  Constant1/1 -> Math Function/1, Divide1/2

== system TBS_SIM/Caipriha Airframe1/Aerodynamic Coefficient/Segment2/left wing/DynamicPressure ==
  v : Inport
  Gain1 : Gain  Gain=air_density
  Gain2 : Gain  Gain=0.5
  Gain3 : Gain  Gain=S_seg2
  Math Function : Math  Operator=magnitude^2  SignedPower=on  SaturateOnIntegerOverflow=on
  p : Outport
  wires:
  Gain3/1 -> p/1
  Gain2/1 -> Gain3/1
  Gain1/1 -> Gain2/1
  Math Function/1 -> Gain1/1
  v/1 -> Math Function/1

== system TBS_SIM/Caipriha Airframe1/Aerodynamic Coefficient/Segment2/left wing/wing ==
  Alpha : Inport
  Delta : Inport  Port=2
  airspeed : Inport  Port=3
  AirspeedLookup : PreLookup  BreakpointsData=as  BeginIndexSearchUsingPreviousIndexResult=on  ExtrapMethod=Linear
  AlphaLookup : PreLookup  BreakpointsData=alpha_vec_0  BeginIndexSearchUsingPreviousIndexResult=on  ExtrapMethod=Linear
  CD : Interpolation_n-D  NumberOfTableDimensions=3  Table=ORIGIN_CD  ExtrapMethod=Clip  DiagnosticForOutOfRangeInput=Warning  InternalRulePriority=Speed
      settings: InputPortMap=u0,u1,u2,u3,u4,u5
  CD1 : Interpolation_n-D  NumberOfTableDimensions=3  Table=ORIGIN_CM  ExtrapMethod=Clip  DiagnosticForOutOfRangeInput=Warning  InternalRulePriority=Speed
      settings: InputPortMap=u0,u1,u2,u3,u4,u5
  CL : Interpolation_n-D  NumberOfTableDimensions=3  Table=ORIGIN_CL  ExtrapMethod=Clip  DiagnosticForOutOfRangeInput=Warning  InternalRulePriority=Speed
      settings: InputPortMap=u0,u1,u2,u3,u4,u5
  DeltaLookup : PreLookup  BreakpointsData=ORIGIN_DELTA  BeginIndexSearchUsingPreviousIndexResult=on  ExtrapMethod=Linear
  cl : Outport
  cd : Outport  Port=2
  cm : Outport  Port=3
  wires:
  Alpha/1 -> AlphaLookup/1
  airspeed/1 -> AirspeedLookup/1
  DeltaLookup/1 -> CD1/5, CL/5, CD/5
  DeltaLookup/2 -> CD1/6, CL/6, CD/6
  CL/1 -> cl/1
  AirspeedLookup/1 -> CD1/1, CD/1, CL/1
  AirspeedLookup/2 -> CD1/2, CD/2, CL/2
  AlphaLookup/1 -> CD/3, CD1/3, CL/3
  AlphaLookup/2 -> CD1/4, CD/4, CL/4
  CD/1 -> cd/1
  CD1/1 -> cm/1
  Delta/1 -> DeltaLookup/1

== system TBS_SIM/Caipriha Airframe1/Aerodynamic Coefficient/Segment2/right wing/DynamicPressure ==
  v : Inport
  Gain1 : Gain  Gain=air_density
  Gain2 : Gain  Gain=0.5
  Gain3 : Gain  Gain=S_seg2
  Math Function : Math  Operator=magnitude^2  SignedPower=on  SaturateOnIntegerOverflow=on
  p : Outport
  wires:
  Gain3/1 -> p/1
  Gain2/1 -> Gain3/1
  Gain1/1 -> Gain2/1
  Math Function/1 -> Gain1/1
  v/1 -> Math Function/1

== system TBS_SIM/Caipriha Airframe1/Aerodynamic Coefficient/Segment2/right wing/wing ==
  Alpha : Inport
  Delta : Inport  Port=2
  airspeed : Inport  Port=3
  AirspeedLookup : PreLookup  BreakpointsData=as  BeginIndexSearchUsingPreviousIndexResult=on  ExtrapMethod=Linear
  AlphaLookup : PreLookup  BreakpointsData=alpha_vec_0  BeginIndexSearchUsingPreviousIndexResult=on  ExtrapMethod=Linear
  CD : Interpolation_n-D  NumberOfTableDimensions=3  Table=ORIGIN_CD  ExtrapMethod=Clip  DiagnosticForOutOfRangeInput=Warning  InternalRulePriority=Speed
      settings: InputPortMap=u0,u1,u2,u3,u4,u5
  CD1 : Interpolation_n-D  NumberOfTableDimensions=3  Table=ORIGIN_CM  ExtrapMethod=Clip  DiagnosticForOutOfRangeInput=Warning  InternalRulePriority=Speed
      settings: InputPortMap=u0,u1,u2,u3,u4,u5
  CL : Interpolation_n-D  NumberOfTableDimensions=3  Table=ORIGIN_CL  ExtrapMethod=Clip  DiagnosticForOutOfRangeInput=Warning  InternalRulePriority=Speed
      settings: InputPortMap=u0,u1,u2,u3,u4,u5
  DeltaLookup : PreLookup  BreakpointsData=ORIGIN_DELTA  BeginIndexSearchUsingPreviousIndexResult=on  ExtrapMethod=Linear
  cl : Outport
  cd : Outport  Port=2
  cm : Outport  Port=3
  wires:
  Alpha/1 -> AlphaLookup/1
  airspeed/1 -> AirspeedLookup/1
  DeltaLookup/1 -> CD1/5, CL/5, CD/5
  DeltaLookup/2 -> CD1/6, CL/6, CD/6
  CL/1 -> cl/1
  AirspeedLookup/1 -> CD1/1, CD/1, CL/1
  AirspeedLookup/2 -> CD1/2, CD/2, CL/2
  AlphaLookup/1 -> CD/3, CD1/3, CL/3
  AlphaLookup/2 -> CD1/4, CD/4, CL/4
  CD/1 -> cd/1
  CD1/1 -> cm/1
  Delta/1 -> DeltaLookup/1

== system TBS_SIM/Caipriha Airframe1/Aerodynamic Coefficient/Segment3L1/wing/DynamicPressure ==
  v : Inport
  Gain1 : Gain  Gain=air_density
  Gain2 : Gain  Gain=0.5
  Gain3 : Gain  Gain=S_seg3
  Math Function : Math  Operator=magnitude^2  SignedPower=on  SaturateOnIntegerOverflow=on
  p : Outport
  wires:
  Gain3/1 -> p/1
  Gain2/1 -> Gain3/1
  Gain1/1 -> Gain2/1
  Math Function/1 -> Gain1/1
  v/1 -> Math Function/1

== system TBS_SIM/Caipriha Airframe1/Aerodynamic Coefficient/Segment3L1/wing/wing ==
  Alpha : Inport
  Delta : Inport  Port=2
  airspeed : Inport  Port=3
  AirspeedLookup : PreLookup  BreakpointsData=as  BeginIndexSearchUsingPreviousIndexResult=on  ExtrapMethod=Linear
  AlphaLookup : PreLookup  BreakpointsData=alpha_vec_0  BeginIndexSearchUsingPreviousIndexResult=on  ExtrapMethod=Linear
  CD : Interpolation_n-D  NumberOfTableDimensions=3  Table=ORIGIN_CD  ExtrapMethod=Clip  DiagnosticForOutOfRangeInput=Warning  InternalRulePriority=Speed
      settings: InputPortMap=u0,u1,u2,u3,u4,u5
  CD1 : Interpolation_n-D  NumberOfTableDimensions=3  Table=ORIGIN_CM  ExtrapMethod=Clip  DiagnosticForOutOfRangeInput=Warning  InternalRulePriority=Speed
      settings: InputPortMap=u0,u1,u2,u3,u4,u5
  CL : Interpolation_n-D  NumberOfTableDimensions=3  Table=ORIGIN_CL  ExtrapMethod=Clip  DiagnosticForOutOfRangeInput=Warning  InternalRulePriority=Speed
      settings: InputPortMap=u0,u1,u2,u3,u4,u5
  DeltaLookup : PreLookup  BreakpointsData=ORIGIN_DELTA  BeginIndexSearchUsingPreviousIndexResult=on  ExtrapMethod=Linear
  cl : Outport
  cd : Outport  Port=2
  cm : Outport  Port=3
  wires:
  Alpha/1 -> AlphaLookup/1
  airspeed/1 -> AirspeedLookup/1
  DeltaLookup/1 -> CD1/5, CL/5, CD/5
  DeltaLookup/2 -> CD1/6, CL/6, CD/6
  CL/1 -> cl/1
  AirspeedLookup/1 -> CD1/1, CD/1, CL/1
  AirspeedLookup/2 -> CD1/2, CD/2, CL/2
  AlphaLookup/1 -> CD/3, CD1/3, CL/3
  AlphaLookup/2 -> CD1/4, CD/4, CL/4
  CD/1 -> cd/1
  CD1/1 -> cm/1
  Delta/1 -> DeltaLookup/1

== system TBS_SIM/Caipriha Airframe1/Aerodynamic Coefficient/Segment3R/right wing/DynamicPressure ==
  v : Inport
  Gain1 : Gain  Gain=air_density
  Gain2 : Gain  Gain=0.5
  Gain3 : Gain  Gain=S_seg3
  Math Function : Math  Operator=magnitude^2  SignedPower=on  SaturateOnIntegerOverflow=on
  p : Outport
  wires:
  Gain3/1 -> p/1
  Gain2/1 -> Gain3/1
  Gain1/1 -> Gain2/1
  Math Function/1 -> Gain1/1
  v/1 -> Math Function/1

== system TBS_SIM/Caipriha Airframe1/Aerodynamic Coefficient/Segment3R/right wing/wing ==
  Alpha : Inport
  Delta : Inport  Port=2
  airspeed : Inport  Port=3
  AirspeedLookup : PreLookup  BreakpointsData=as  BeginIndexSearchUsingPreviousIndexResult=on  ExtrapMethod=Linear
  AlphaLookup : PreLookup  BreakpointsData=alpha_vec_0  BeginIndexSearchUsingPreviousIndexResult=on  ExtrapMethod=Linear
  CD : Interpolation_n-D  NumberOfTableDimensions=3  Table=ORIGIN_CD  ExtrapMethod=Clip  DiagnosticForOutOfRangeInput=Warning  InternalRulePriority=Speed
      settings: InputPortMap=u0,u1,u2,u3,u4,u5
  CD1 : Interpolation_n-D  NumberOfTableDimensions=3  Table=ORIGIN_CM  ExtrapMethod=Clip  DiagnosticForOutOfRangeInput=Warning  InternalRulePriority=Speed
      settings: InputPortMap=u0,u1,u2,u3,u4,u5
  CL : Interpolation_n-D  NumberOfTableDimensions=3  Table=ORIGIN_CL  ExtrapMethod=Clip  DiagnosticForOutOfRangeInput=Warning  InternalRulePriority=Speed
      settings: InputPortMap=u0,u1,u2,u3,u4,u5
  DeltaLookup : PreLookup  BreakpointsData=ORIGIN_DELTA  BeginIndexSearchUsingPreviousIndexResult=on  ExtrapMethod=Linear
  cl : Outport
  cd : Outport  Port=2
  cm : Outport  Port=3
  wires:
  Alpha/1 -> AlphaLookup/1
  airspeed/1 -> AirspeedLookup/1
  DeltaLookup/1 -> CD1/5, CL/5, CD/5
  DeltaLookup/2 -> CD1/6, CL/6, CD/6
  CL/1 -> cl/1
  AirspeedLookup/1 -> CD1/1, CD/1, CL/1
  AirspeedLookup/2 -> CD1/2, CD/2, CL/2
  AlphaLookup/1 -> CD/3, CD1/3, CL/3
  AlphaLookup/2 -> CD1/4, CD/4, CL/4
  CD/1 -> cd/1
  CD1/1 -> cm/1
  Delta/1 -> DeltaLookup/1
